simulink model "Encoder_reader_simulink"  (R2025a)
settings: Solver=FixedStepAuto  StartTime=0.0  StopTime=100  FixedStep=0.01  RelTol=1e-3  EnableMultiTasking=on
libraries: stm32g4xxblockslib x3, stm32f4xxblockslib x2
settings Model: STM32="{\"EncoderBlockForG4\":[{\"ID\":\"untitled:1\"},{\"ID\":\"Lab3_Encoder:1\"},{\"ID\":\"Encoder_reader_simulink:1\"},{\"ID\":\"Encoder_reader_simulink:50\"},{\"ID\":\"Encoder_reader_simulink:51\"}],\"DigitalPortRead\":[{\"ID\":\"Encoder_reader_simulink:53\"},{\"ID\":\"Encoder_reader_simulink:54\"}]}"  Creator=User  LastModifiedBy=POND
settings OptimizationCC: DefaultParameterBehavior=Inlined  EnhancedBackFolding=on  PassReuseOutputArgsAs=Individual arguments  ZeroExternalMemoryAtStartup=off  ZeroInternalMemoryAtStartup=off  MaxStackSize=512  OptimizeBlockOrder=speed  DifferentSizesBufferReuse=on  OptimizationCustomize=off  EfficientTunableParamExpr=on
settings DebuggingCC: ParameterTunabilityLossMsg=error
settings HardwareCC: ProdBitPerPointer=32.0  ProdBitPerSizeT=32.0  ProdBitPerPtrDiffT=32.0  ProdLargestAtomicInteger=Long  ProdLargestAtomicFloat=Double  ProdWordSize=32.0  ProdLongLongMode=on  ProdHWDeviceType=ARM Compatible->ARM Cortex-M
settings SFSimCC: MATLABDynamicMemAlloc=off
settings RTWCC: SystemTargetFile=ert.tlc  HardwareBoard=STM32G4xx Based  TemplateMakefile=ert_default_tmf  Toolchain=GNU Tools for ARM Embedded Processors  Description=Embedded Coder
settings CodeAppCC: ForceParamTrailComments=on  IgnoreCustomStorageClasses=off  OperatorAnnotations=on  SimulinkDataObjDesc=on  SFDataObjDesc=on  InsertBlockDesc=on
settings ERTTargetCC: ExtModeTransport=3.0  ExtModeStaticAllocSize=2048.0  TargetLangStandard=C99 (ISO)  CodeReplacementLibrary=ARM Cortex-M  SupportContinuousTime=on

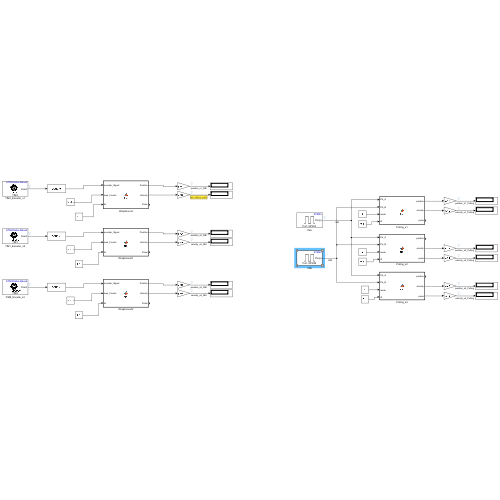
[thumbnail: Simulink's stored preview of the top-level diagram]
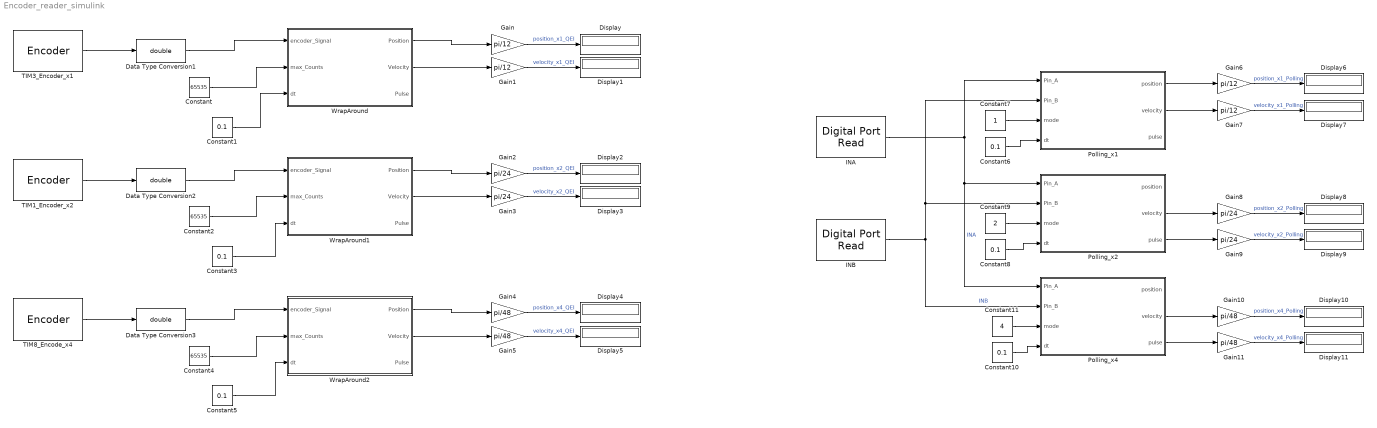
== system Encoder_reader_simulink ==
  Constant : Constant  Value=65535
  Constant{1,3,5..6,8,10} (6 alike) : Constant  Value=0.1
  Constant11 : Constant  Value=4
  Constant2 : Constant  Value=65535
  Constant4 : Constant  Value=65535
  Constant7 : Constant
  Constant9 : Constant  Value=2
  Data Type Conversion1 : DataTypeConversion  OutDataTypeStr=double  SaturateOnIntegerOverflow=off  RndMeth=Floor
  Data Type Conversion2 : DataTypeConversion  OutDataTypeStr=double  SaturateOnIntegerOverflow=off  RndMeth=Floor
  Data Type Conversion3 : DataTypeConversion  OutDataTypeStr=double  SaturateOnIntegerOverflow=off  RndMeth=Floor
  Display{,1..11} (12 alike) : Display
  Gain{,1,6..7} (4 alike) : Gain  Gain=pi/12
  Gain{4..5,10..11} (4 alike) : Gain  Gain=pi/48
  Gain{2..3,8..9} (4 alike) : Gain  Gain=pi/24
  INA : stm32f4xxblockslib/Digital Port Read  PortName=GPIOA  PinNumber=[8]  ReadOperation=on  IOAsArray=on  SampleTime=-1  EnableSimPort=off  hoistedMaskSrc=ECSoC/ECSimCodegen/Digital Port Read
      settings: LibrarySourceBlock=stm32g4xxblockslib/Digital Port Read
  INB : stm32f4xxblockslib/Digital Port Read  PortName=GPIOB  PinNumber=[10]  ReadOperation=on  IOAsArray=on  SampleTime=-1  EnableSimPort=off  hoistedMaskSrc=ECSoC/ECSimCodegen/Digital Port Read
      settings: LibrarySourceBlock=stm32g4xxblockslib/Digital Port Read
  Polling_x1 : MATLAB Function  TreatAsAtomicUnit=on
  Polling_x2 : MATLAB Function  TreatAsAtomicUnit=on
  Polling_x4 : MATLAB Function  TreatAsAtomicUnit=on
  TIM1_Encoder_x2 : stm32g4xxblockslib/Encoder  TimerModule=TIM1  EnableResetInput=off  OutputCountAfterFirstIndex=off  OutputValidIndex=off  OutputDirection=off  OutputStatus=off  SampleTime=-1
  TIM3_Encoder_x1 : stm32g4xxblockslib/Encoder  TimerModule=TIM3  EnableResetInput=off  OutputCountAfterFirstIndex=off  OutputValidIndex=off  OutputDirection=off  OutputStatus=off  SampleTime=-1
  TIM8_Encode_x4 : stm32g4xxblockslib/Encoder  TimerModule=TIM8  EnableResetInput=off  OutputCountAfterFirstIndex=off  OutputValidIndex=off  OutputDirection=off  OutputStatus=off  SampleTime=-1
  WrapAround : MATLAB Function  TreatAsAtomicUnit=on
  WrapAround1 : MATLAB Function  TreatAsAtomicUnit=on
  WrapAround2 : MATLAB Function  TreatAsAtomicUnit=on
  wires:
  TIM3_Encoder_x1/1 -> Data Type Conversion1/1
  Data Type Conversion1/1 -> WrapAround/1(encoder_Signal)
  Constant/1 -> WrapAround/2(max_Counts)
  WrapAround/1(Position) -> Gain/1
  WrapAround/2(Velocity) -> Gain1/1
  Gain1/1 -> Display1/1  "velocity_x1_QEI"
  Gain/1 -> Display/1  "position_x1_QEI"
  Constant2/1 -> WrapAround1/2(max_Counts)
  Constant3/1 -> WrapAround1/3(dt)
  WrapAround1/1(Position) -> Gain2/1
  Gain3/1 -> Display3/1  "velocity_x2_QEI"
  WrapAround1/2(Velocity) -> Gain3/1
  TIM1_Encoder_x2/1 -> Data Type Conversion2/1
  Data Type Conversion2/1 -> WrapAround1/1(encoder_Signal)
  Gain2/1 -> Display2/1  "position_x2_QEI"
  Constant4/1 -> WrapAround2/2(max_Counts)
  Constant5/1 -> WrapAround2/3(dt)
  WrapAround2/1(Position) -> Gain4/1
  Gain5/1 -> Display5/1  "velocity_x4_QEI"
  WrapAround2/2(Velocity) -> Gain5/1
  TIM8_Encode_x4/1 -> Data Type Conversion3/1
  Data Type Conversion3/1 -> WrapAround2/1(encoder_Signal)
  Gain4/1 -> Display4/1  "position_x4_QEI"
  Constant1/1 -> WrapAround/3(dt)
  INA/1 -> Polling_x1/1(Pin_A), Polling_x4/1(Pin_A), Polling_x2/1(Pin_A)  "INA"
  INB/1 -> Polling_x4/2(Pin_B), Polling_x2/2(Pin_B), Polling_x1/2(Pin_B)  "INB"
  Constant6/1 -> Polling_x1/4(dt)
  Constant7/1 -> Polling_x1/3(mode)
  Constant9/1 -> Polling_x2/3(mode)
  Constant8/1 -> Polling_x2/4(dt)
  Constant11/1 -> Polling_x4/3(mode)
  Constant10/1 -> Polling_x4/4(dt)
  Gain8/1 -> Display8/1  "position_x2_Polling"
  Gain6/1 -> Display6/1  "position_x1_Polling"
  Gain10/1 -> Display10/1  "position_x4_Polling"
  Gain11/1 -> Display11/1  "velocity_x4_Polling"
  Gain9/1 -> Display9/1  "velocity_x2_Polling"
  Gain7/1 -> Display7/1  "velocity_x1_Polling"
  Polling_x1/1(position) -> Gain6/1
  Polling_x1/2(velocity) -> Gain7/1
  Polling_x2/2(velocity) -> Gain8/1
  Polling_x2/3(pulse) -> Gain9/1
  Polling_x4/2(velocity) -> Gain10/1
  Polling_x4/3(pulse) -> Gain11/1

== matlab function Encoder_reader_simulink/WrapAround1 ==
  data: encoder_Signal input; Position output; max_Counts input; Velocity output; Pulse output; dt input
function [Position, Velocity, Pulse] = fcn(encoder_Signal, max_Counts, dt)
    
    persistent prev_Signal corrected_Sum;

    if isempty(prev_Signal)
        prev_Signal = encoder_Signal;
        corrected_Sum = double(encoder_Signal); 
    end

    encoder_Signal = double(encoder_Signal);
    prev_Signal = double(prev_Signal);
    max_Counts = double(max_Counts);
    
    delta = encoder_Signal - prev_Signal;
    

    if delta < -max_Counts/2

        corrected_delta = delta + max_Counts;
    elseif delta > max_Counts/2

        corrected_delta = delta - max_Counts;
    else

        corrected_delta = delta;
    end
    
    corrected_Sum = corrected_Sum + corrected_delta;

    if dt > 0
        Velocity = corrected_delta / dt;
    else
        Velocity = 0;
    end


    prev_Signal = encoder_Signal; 
    Position = corrected_Sum;
    Pulse = encoder_Signal; 
end

== matlab function Encoder_reader_simulink/WrapAround ==
  data: encoder_Signal input; Position output; max_Counts input; Velocity output; Pulse output; dt input
function [Position, Velocity, Pulse] = fcn(encoder_Signal, max_Counts, dt)
    
    persistent prev_Signal corrected_Sum;

    if isempty(prev_Signal)
        prev_Signal = encoder_Signal;
        corrected_Sum = double(encoder_Signal); % Use double for large sums
    end

 
    encoder_Signal = double(encoder_Signal);
    prev_Signal = double(prev_Signal);
    max_Counts = double(max_Counts);
    
    delta = encoder_Signal - prev_Signal;
    

    if delta < -max_Counts/2
      
        corrected_delta = delta + max_Counts;
    elseif delta > max_Counts/2
      
        corrected_delta = delta - max_Counts;
    else
      
        corrected_delta = delta;
    end
    
  
    corrected_Sum = corrected_Sum + corrected_delta;

   
    if dt > 0
        Velocity = corrected_delta / dt;
    else
        Velocity = 0;
    end


    prev_Signal = encoder_Signal;
    Position = corrected_Sum;
    Pulse = encoder_Signal;
end

== matlab function Encoder_reader_simulink/WrapAround2 ==
  data: encoder_Signal input; Position output; max_Counts input; Velocity output; Pulse output; dt input
% Add 'dt' as a new input to your function block
function [Position, Velocity, Pulse] = fcn(encoder_Signal, max_Counts, dt)
    
    persistent prev_Signal corrected_Sum;

    if isempty(prev_Signal)
        prev_Signal = encoder_Signal;
        corrected_Sum = double(encoder_Signal); % Use double for large sums
    end

    % --- Convert inputs to double for correct math ---
    encoder_Signal = double(encoder_Signal);
    prev_Signal = double(prev_Signal);
    max_Counts = double(max_Counts);
    
    delta = encoder_Signal - prev_Signal;
    
    % --- 1. Handle Counter Unwrapping ---
    if delta < -max_Counts/2
        % Overflow (e.g., 65535 -> 1)
        corrected_delta = delta + max_Counts;
    elseif delta > max_Counts/2
        % Underflow (e.g., 1 -> 65535)
        corrected_delta = delta - max_Counts;
    else
        % No wrap
        corrected_delta = delta;
    end
    
    % Add the *corrected* change to the total sum
    corrected_Sum = corrected_Sum + corrected_delta;

    % --- 2. Calculate Velocity (using the corrected delta) ---
    if dt > 0
        Velocity = corrected_delta / dt;
    else
        Velocity = 0; % Avoid division by zero
    end

    % --- 3. Update memory and set outputs ---
    prev_Signal = encoder_Signal; % Save current value for next time
    Position = corrected_Sum;
    Pulse = encoder_Signal; % Pass through the raw signal
end

== matlab function Encoder_reader_simulink/Polling_x1 ==
  data: Pin_A input; position output; Pin_B input; mode input; velocity output; pulse output; dt input
% Function fcn(Pin_A, Pin_B, mode, dt)
% This function combines x1, x2, and x4 software polling logic.
function [position, velocity, pulse] = fcn(Pin_A, Pin_B, mode, dt)

    % --- Persistent variables to store state ---
    % These are local to THIS block instance
    persistent last_A last_B pos;
    persistent lookup_table; % Only used by x4
 
    % --- First-time initialization ---
    if isempty(pos)
        last_A = Pin_A;
        last_B = Pin_B;
        pos = int32(0); 
        
        % Initialize the x4 lookup table (it's fine if unused)
        % [last_A, last_B, curr_A, curr_B]
        lookup_table = int8([0, -1, 1, 0, 1, 0, 0, -1, -1, 0, 0, 1, 0, 1, -1, 0]);
    end

    change = int32(0); % Default change is 0

    % --- Select logic based on 'mode' input ---
    switch mode
        case 1
            % --- x1 Logic: Rising Edge of A ---
            if Pin_A == true && last_A == false
                if Pin_B == false
                    change = int32(1); % CW
                else
                    change = int32(-1); % CCW
                end
            end
        
        case 2
            % --- x2 Logic: Any Edge of A ---
            if Pin_A ~= last_A
                if Pin_A ~= Pin_B
                    change = int32(1); % CW
                else
                    change = int32(-1); % CCW
                end
            end

        case 4
            % --- x4 Logic: Lookup Table (Any Edge of A or B) ---
            last_A_uint = uint8(last_A);
            last_B_uint = uint8(last_B);
            Pin_A_uint = uint8(Pin_A);
            Pin_B_uint = uint8(Pin_B);

            index = bitshift(last_A_uint, 3) | bitshift(last_B_uint, 2) | bitshift(Pin_A_uint, 1) | Pin_B_uint;
            change = int32(lookup_table(index + 1));
        
        otherwise
            % If mode is not 1, 2, or 4, do nothing
            change = int32(0);
    end
 
    % --- Update Position ---
    pos = pos + change;
 
    % --- Calculate Velocity ---
    if dt > 0
        velocity = double(change) / dt;
    else
        velocity = 0.0;
    end
 
    % --- Update states and set outputs ---
    last_A = Pin_A;
    last_B = Pin_B;
    position = pos;
    pulse = Pin_A; % Output Pin A status
end

== matlab function Encoder_reader_simulink/Polling_x2 ==
  data: Pin_A input; position output; Pin_B input; mode input; velocity output; pulse output; dt input

function [position, velocity, pulse] = fcn(Pin_A, Pin_B, mode, dt)


    persistent last_A last_B pos;
    persistent lookup_table;

    if isempty(pos)
        last_A = Pin_A;
        last_B = Pin_B;
        pos = int32(0); 
        
        lookup_table = int8([0, -1, 1, 0, 1, 0, 0, -1, -1, 0, 0, 1, 0, 1, -1, 0]);
    end

    change = int32(0);


    switch mode
        case 1
 
            if Pin_A == true && last_A == false
                if Pin_B == false
                    change = int32(1); % CW
                else
                    change = int32(-1); % CCW
                end
            end
        
        case 2

            if Pin_A ~= last_A
                if Pin_A ~= Pin_B
                    change = int32(1); % CW
                else
                    change = int32(-1); % CCW
                end
            end

        case 4

            last_A_uint = uint8(last_A);
            last_B_uint = uint8(last_B);
            Pin_A_uint = uint8(Pin_A);
            Pin_B_uint = uint8(Pin_B);

            index = bitshift(last_A_uint, 3) | bitshift(last_B_uint, 2) | bitshift(Pin_A_uint, 1) | Pin_B_uint;
            change = int32(lookup_table(index + 1));
        
        otherwise

            change = int32(0);
    end
 

    pos = pos + change;
 

    if dt > 0
        velocity = double(change) / dt;
    else
        velocity = 0.0;
    end
 
    last_A = Pin_A;
    last_B = Pin_B;
    position = pos;
    pulse = Pin_A; % Output Pin A status
end

== matlab function Encoder_reader_simulink/Polling_x4 ==
  data: Pin_A input; position output; Pin_B input; mode input; velocity output; pulse output; dt input
% Function fcn(Pin_A, Pin_B, mode, dt)
% This function combines x1, x2, and x4 software polling logic.
function [position, velocity, pulse] = fcn(Pin_A, Pin_B, mode, dt)

    % --- Persistent variables to store state ---
    % These are local to THIS block instance
    persistent last_A last_B pos;
    persistent lookup_table; % Only used by x4
 
    % --- First-time initialization ---
    if isempty(pos)
        last_A = Pin_A;
        last_B = Pin_B;
        pos = int32(0); 
        
        % Initialize the x4 lookup table (it's fine if unused)
        % [last_A, last_B, curr_A, curr_B]
        lookup_table = int8([0, -1, 1, 0, 1, 0, 0, -1, -1, 0, 0, 1, 0, 1, -1, 0]);
    end

    change = int32(0); % Default change is 0

    % --- Select logic based on 'mode' input ---
    switch mode
        case 1
            % --- x1 Logic: Rising Edge of A ---
            if Pin_A == true && last_A == false
                if Pin_B == false
                    change = int32(1); % CW
                else
                    change = int32(-1); % CCW
                end
            end
        
        case 2
            % --- x2 Logic: Any Edge of A ---
            if Pin_A ~= last_A
                if Pin_A ~= Pin_B
                    change = int32(1); % CW
                else
                    change = int32(-1); % CCW
                end
            end

        case 4
            % --- x4 Logic: Lookup Table (Any Edge of A or B) ---
            last_A_uint = uint8(last_A);
            last_B_uint = uint8(last_B);
            Pin_A_uint = uint8(Pin_A);
            Pin_B_uint = uint8(Pin_B);

            index = bitshift(last_A_uint, 3) | bitshift(last_B_uint, 2) | bitshift(Pin_A_uint, 1) | Pin_B_uint;
            change = int32(lookup_table(index + 1));
        
        otherwise
            % If mode is not 1, 2, or 4, do nothing
            change = int32(0);
    end
 
    % --- Update Position ---
    pos = pos + change;
 
    % --- Calculate Velocity ---
    if dt > 0
        velocity = double(change) / dt;
    else
        velocity = 0.0;
    end
 
    % --- Update states and set outputs ---
    last_A = Pin_A;
    last_B = Pin_B;
    position = pos;
    pulse = Pin_A; % Output Pin A status
end
